simulink model "reaction_wheel"  (R2015a)
settings: Solver=FixedStepDiscrete  StartTime=0.0  StopTime=10.0  FixedStep=delta_t  RelTol=1e-3
undefined symbols (not defined in the file): D, delta_t
settings Model: Creator=Kerianne  LastModifiedBy=Kerianne
settings DataIOCC: SaveFormat=Structure
settings OptimizationCC: InlineParams=on  ExpressionDepthLimit=2147483647
settings DebuggingCC: UnderspecifiedInitializationDetection=Classic  MergeDetectMultiDrivingBlocksExec=none  SolverPrmCheckMsg=warning  StateNameClashWarn=warning

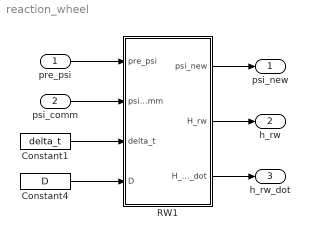
== system reaction_wheel ==
  pre_psi : Inport
  psi_comm : Inport  Port=2
  Constant1 : Constant  Value=delta_t
  Constant4 : Constant  Value=D
  RW1 : MATLAB Function  TreatAsAtomicUnit=on
  psi_new : Outport
  h_rw : Outport  Port=2
  h_rw_dot : Outport  Port=3
  wires:
  RW1/1(psi_new) -> psi_new/1
  Constant4/1 -> RW1/4(D)
  pre_psi/1 -> RW1/1(pre_psi)
  psi_comm/1 -> RW1/2(psi_dot_comm)
  Constant1/1 -> RW1/3(delta_t)
  RW1/2(H_rw) -> h_rw/1
  RW1/3(H_rw_dot) -> h_rw_dot/1

== matlab function reaction_wheel/RW1 ==
  data: pre_psi input; psi_dot_comm input; delta_t input; psi_new output; H_rw output; H_rw_dot output; D input
function  [psi_new,H_rw,H_rw_dot]= fcn(pre_psi, psi_dot_comm, delta_t,D)
% Reaction Wheel Dynamics
% Author: Kerianne Gross, AFRL/RQQA, kerianne.gross@us.af.mil
% Last Updated: 5 May 2015 

% set acceleration to commanded acceleration
psi_dot = psi_dot_comm;
% calculate change in angular momentum contribution
H_rw_dot = D*psi_dot;   
% calculate new angular velocity
psi_new = pre_psi + psi_dot*delta_t;  
% calculate change in angular momentum contribution
H_rw = D*psi_new;
